simulink model "Td2Microc"  (R2017b)
settings: Solver=ode23t  StartTime=0.0  StopTime=0.5  RelTol=1e-3
InitFcn:
  | Td2
values from neighbouring files (symbols this model uses):
  b = 3.5077E-6    (= 3.5077e-06)    [MCC_constants.m]    (also in Td2.m = 0.0085; Tp3_data.m = 0.0085)
  Cr = 0    [MCC_constants.m]    (also in Td2.m; Tp3_data.m)
  J = 3.2284E-6    (= 3.2284e-06)    [MCC_constants.m]    (also in ProjetGiesData.m = 0.5; Td2.m = 0.28; Tp3_data.m = 0.2)
  K = 0.0274    [MCC_constants.m]    (also in Td2.m = 0.5093; Tp3_data.m = 0.9)
  Kp = 1.125    [Td2.m]    (also in Tp3_data.m = 1)
  L = 2.75E-6    (= 2.75e-06)    [MCC_constants.m]    (also in Td2.m = 0.0016; Tp3_data.m = 0.012161)
  R = 4    [MCC_constants.m]    (also in Td2.m = 0.13; Tp3_data.m = 0.895)
libraries: simulink x2
settings Model: Creator=Table2  LastModifiedBy=Table2

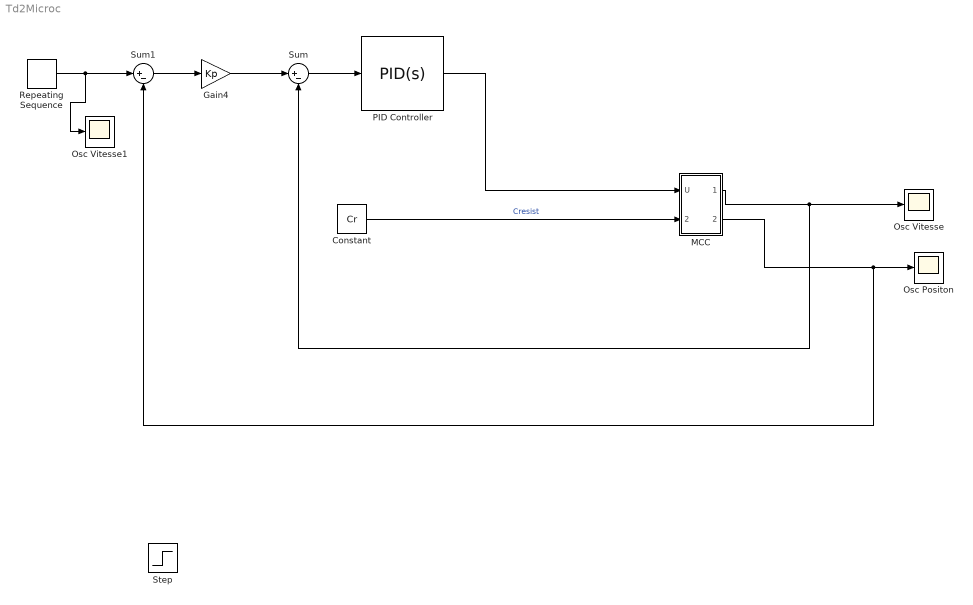
== system Td2Microc ==
  Constant : Constant  Value=Cr
  Gain4 : Gain  Gain=Kp
  MCC : Subsystem
  Osc Positon : Scope
  Osc Vitesse : Scope
  Osc Vitesse1 : Scope
  PID Controller : simulink/Continuous/PID Controller  Controller=PID  TimeDomain=Continuous-time  SampleTime=-1  IntegratorMethod=Forward Euler  FilterMethod=Forward Euler  Form=Parallel  UseFilter=on  ControllerParametersSource=internal  P=3  I=40  D=0.035  N=100  InitialConditionSource=internal  InitialConditionForIntegrator=0  InitialConditionForFilter=0  ExternalReset=none  LimitOutput=off  UpperSaturationLimit=inf  LowerSaturationLimit=-inf  LinearizeAsGain=on  AntiWindupMode=none  Kb=1  TrackingMode=off  Kt=1  PParamMin=[]  PParamMax=[]  IParamMin=[]  IParamMax=[]  DParamMin=[]  DParamMax=[]  NParamMin=[]  NParamMax=[]  KbParamMin=[]  KbParamMax=[]  KtParamMin=[]  KtParamMax=[]  POutMin=[]  POutMax=[]  IOutMin=[]  IOutMax=[]  DOutMin=[]  DOutMax=[]  NOutMin=[]  NOutMax=[]  KbOutMin=[]  KbOutMax=[]  KtOutMin=[]  KtOutMax=[]  IntegratorOutMin=[]  IntegratorOutMax=[]  FilterOutMin=[]  FilterOutMax=[]  SumOutMin=[]  SumOutMax=[]  SumI1OutMin=[]  SumI1OutMax=[]  SumI2OutMin=[]  SumI2OutMax=[]  SumI3OutMin=[]  SumI3OutMax=[]  SumDOutMin=[]  SumDOutMax=[]  SaturationOutMin=[]  SaturationOutMax=[]  IntegratorContinuousStateAttributes=''  IntegratorStateMustResolveToSignalObject=off  IntegratorRTWStateStorageClass=Auto  FilterContinuousStateAttributes=''  FilterStateMustResolveToSignalObject=off  FilterRTWStateStorageClass=Auto  DifferentiatorICPrevScaledInput=0  DifferentiatorOutMin=[]  DifferentiatorOutMax=[]  InitialConditionSetting=State (most efficient)  FilterDiffOutCoefMin=[]  FilterDiffOutCoefMax=[]  SumDenOutMin=[]  SumDenOutMax=[]  SumNumOutMin=[]  SumNumOutMax=[]  ReciprocalOutMin=[]  ReciprocalOutMax=[]  DivideOutMin=[]  DivideOutMax=[]  TunerSelectOption=Transfer Function Based (PID Tuner App)
  Repeating Sequence : simulink/Sources/Repeating Sequence  rep_seq_t=[0 0.1 0.2 0.3 1]  rep_seq_y=[0 50 50 0 0.]
  Step : Step  Time=0  SampleTime=0
  Sum : Sum  Inputs=|+-
  Sum1 : Sum  Inputs=|+-
  wires:
  Constant/1 -> MCC/2(In2)  "Cresist"
  MCC/1(Out1) -> Sum/2, Osc Vitesse/1
  Sum/1 -> PID Controller/1
  PID Controller/1 -> MCC/1(U)
  Sum1/1 -> Gain4/1
  Gain4/1 -> Sum/1
  MCC/2(Out2) -> Sum1/2, Osc Positon/1
  Repeating Sequence/1 -> Osc Vitesse1/1, Sum1/1

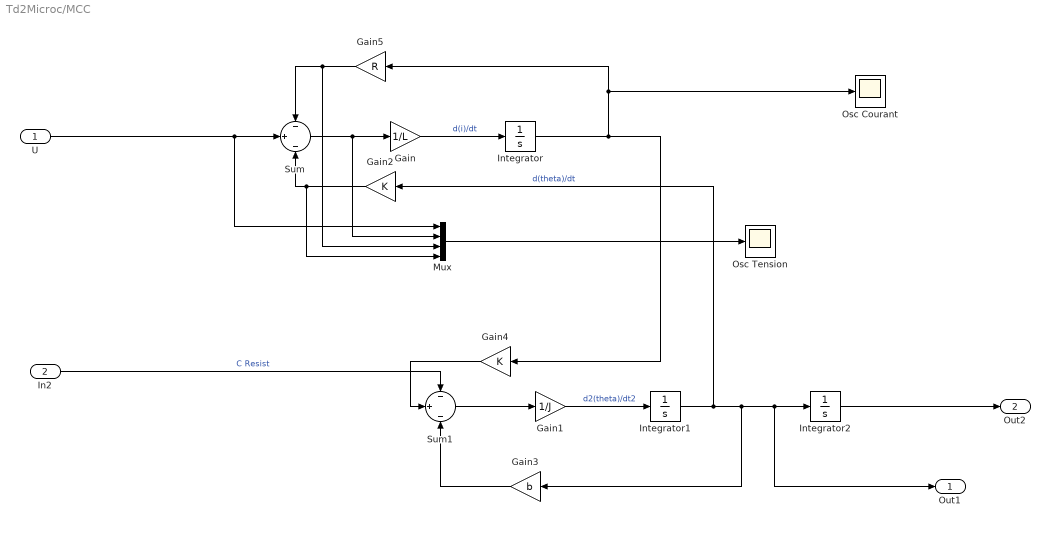
== system Td2Microc/MCC ==
  U : Inport
  In2 : Inport  Port=2
  Gain : Gain  Gain=1/L
  Gain1 : Gain  Gain=1/J
  Gain2 : Gain  Gain=K
  Gain3 : Gain  Gain=b
  Gain4 : Gain  Gain=K
  Gain5 : Gain  Gain=R
  Integrator : Integrator
  Integrator1 : Integrator
  Integrator2 : Integrator
  Mux : Mux
  "Osc Courant " : Scope
  Osc Tension : Scope
  Sum : Sum  Inputs=-|+|-
  Sum1 : Sum  Inputs=-|+|-
  Out1 : Outport
  Out2 : Outport  Port=2
  wires:
  Gain4/1 -> Sum1/2
  Gain3/1 -> Sum1/3
  Gain2/1 -> Mux/4, Sum/3
  Gain5/1 -> Mux/3, Sum/1
  In2/1 -> Sum1/1  "C Resist"
  Integrator/1 -> "Osc Courant "/1, Gain5/1, Gain4/1
  Sum1/1 -> Gain1/1
  Gain1/1 -> Integrator1/1  "d2(theta)/dt2"
  Integrator1/1 -> Gain2/1, Out1/1, Integrator2/1, Gain3/1  "d(theta)/dt"
  Mux/1 -> Osc Tension/1
  Sum/1 -> Mux/2, Gain/1
  U/1 -> Mux/1, Sum/2
  Gain/1 -> Integrator/1  "d(i)/dt"
  Integrator2/1 -> Out2/1
